simulink model "controller_AWBT_implementation"  (Simulink 7.1)
settings: Solver=ode5  StartTime=0.0  StopTime=9  FixedStep=1e-4  RelTol=1e-3
values from neighbouring files (symbols this model uses):
  Ap = A    [main_matlab_version_4.m]    (also in plant.mat = [-0.773996386153 -96.4009703983 0 0 96.979553948 -1.63547954)
  Bp = B    [main_matlab_version_4.m]    (also in plant.mat = [-0.230745598618  -0.153904745996; 0.0612777559553  0.060617)
  Cp = C    [main_matlab_version_4.m]    (also in plant.mat = [-23.1554338545 9.56281796835 0.435674513054 -0.46619419818])
  Hp = E    [main_matlab_version_4.m]    (also in plant.mat = [0.258916103899 0.10195659276 -1.80129126805 -4.56185147008])
  Lambda = [5.58858586263e-05  0.000107348957209; 5.1607851515e-05  9.34227642014e-05; -0.000303330434435  -0.000279469710906; -0.00200633369332  -0.00367108921652; -0.999913291495  0.000114263611536; 0.000204848209343  -0.999721959339]    [controller_khat.mat]
libraries: simulink x1, cstblocks x1
settings Model: Creator=p4wp4w  LastModifiedBy=p4wp4w
settings SolverCC: AlgebraicLoopSolver=LineSearch
settings OptimizationCC: ExpressionDepthLimit=128  InitFltsAndDblsToZero=off
settings DebuggingCC: SolverPrmCheckMsg=none  FcnCallInpInsideContextMsg=Enable All  StateNameClashWarn=none  StrictBusMsg=ErrorLevel1
settings CodeAppCC: CustomSymbolStrType=$N$R$M_T
settings GRTTargetCC: TargetFunctionLibrary=C89/C90 (ANSI)  CPPClassGenCompliant=off

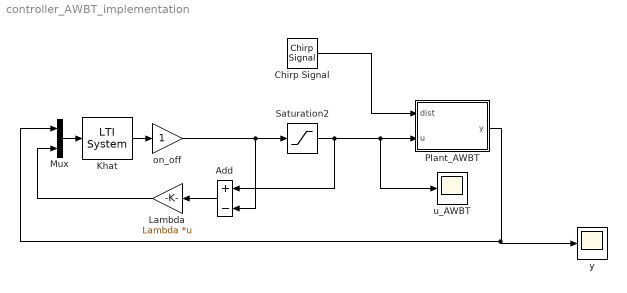
== system controller_AWBT_implementation ==
  Add : Sum  Orientation=left  Inputs=+-
  Chirp Signal : simulink/Sources/Chirp Signal  f1=0.1  T=9  f2=90
  Khat : cstblocks/LTI System  sys=Khat  IC=[]
  Lambda : Gain  Orientation=left  Gain=Lambda  Multiplication=Matrix(K*u)
  Mux : Mux  Inputs=2
  Plant_AWBT : Subsystem
  Saturation2 : Saturate  UpperLimit=1.5  LowerLimit=-1.5
  on_off : Gain
  u_AWBT : Scope
      settings: YMin=-0.75  YMax=0.75
  y : Scope
  wires:
  Mux/1 -> Khat/1
  Khat/1 -> on_off/1
  on_off/1 -> Add/2, Saturation2/1
  Saturation2/1 -> Add/1, u_AWBT/1, Plant_AWBT/2(u)
  Plant_AWBT/1(y) -> y/1, Mux/1
  Lambda/1 -> Mux/2
  Add/1 -> Lambda/1
  Chirp Signal/1 -> Plant_AWBT/1(dist)

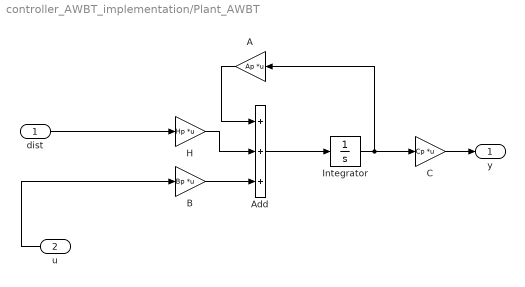
== system controller_AWBT_implementation/Plant_AWBT ==
  dist : Inport
  u : Inport  Orientation=left  Port=2
  A : Gain  Orientation=left  Gain=Ap  Multiplication=Matrix(K*u)
  Add : Sum  Inputs=+++
  B : Gain  Gain=Bp  Multiplication=Matrix(K*u)
  C : Gain  Gain=Cp  Multiplication=Matrix(K*u)
  H : Gain  Gain=Hp  Multiplication=Matrix(K*u)
  Integrator : Integrator
  y : Outport
  wires:
  Add/1 -> Integrator/1
  H/1 -> Add/2
  A/1 -> Add/1
  dist/1 -> H/1
  C/1 -> y/1
  B/1 -> Add/3
  Integrator/1 -> C/1, A/1
  u/1 -> B/1
